simulink model "Linearized_Unicycle_Dynamics_Model"  (R2017b)
settings: Solver=VariableStepAuto  StartTime=0.0  StopTime=10  RelTol=1e-3
settings Model: Creator=Jesus  LastModifiedBy=Jesus

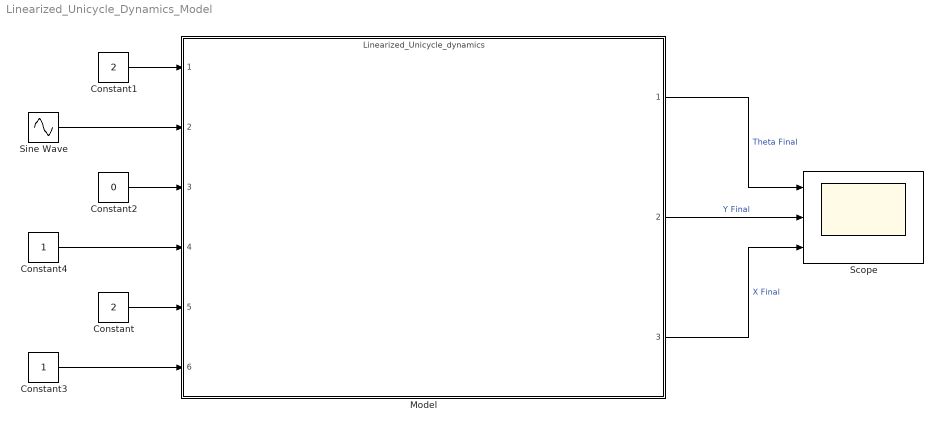
== system Linearized_Unicycle_Dynamics_Model ==
  Constant : Constant  Value=2
  Constant1 : Constant  Value=2
  Constant2 : Constant  Value=0
  Constant3 : Constant
  Constant4 : Constant
  Model : ModelReference  ModelNameDialog=Linearized_Unicycle_dynamics.slx  SimulationMode=Normal  ModelReferenceVersion=1.1
  Scope : Scope  NumInputPorts=3
  Sine Wave : Sin  Frequency=0.01  SampleTime=0
  wires:
  Model/1 -> Scope/1  "Theta Final"
  Model/2 -> Scope/2  "Y Final"
  Model/3 -> Scope/3  "X Final"
  Constant/1 -> Model/5
  Constant1/1 -> Model/1
  Constant2/1 -> Model/3
  Constant3/1 -> Model/6
  Sine Wave/1 -> Model/2
  Constant4/1 -> Model/4
